simulink model "SIL_Microgrid"  (R2024a)
settings: Solver=FixedStepDiscrete  StartTime=0.0  StopTime=10  FixedStep=T_simulation  RelTol=1e-3
model workspace (MAT data in the model file):
  ICAR = 3200
  ICR = 3200
  P_0 = 0
  P_s = 10000
  Q_0 = 0
  Q_s = 1000
  T_f_VI = 0.1
  T_sampleFFR = 0.01
  T_simulation = 0.001
  batteryCellCapacity_Ah = 2
  m_p_VI = 0.1
  numberCellsParallel = 1
  numberCellsSerial = 200
libraries: spsControlledCurrentSourceLib x6, spsThreePhaseVIMeasurementLib x4, spsControlledVoltageSourceLib x3, spsGroundLib x3, spsThreePhaseParallelRLCBranchLib x3, spsThreePhaseSeriesRLCBranchLib x3, eeGeneralControl x2, simulink_extras x2, spsThreePhaseSineGeneratorLib x2, eeSinGeneratorThreePhase x1, eePowerMeasurement x1, sps_lib x1
(part 1 of 2)
settings Model: Creator=Jonathan  LastModifiedBy=Jonathan
settings DebuggingCC: AlgebraicLoopMsg=none

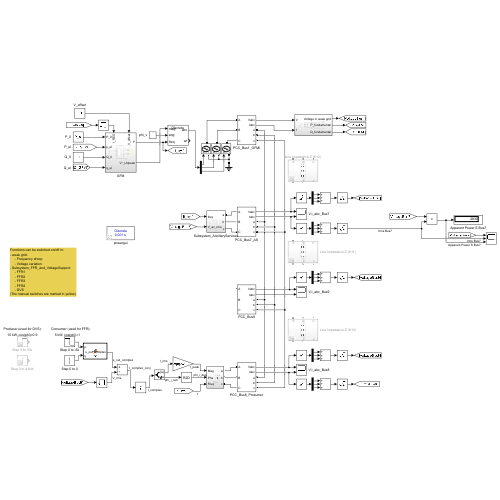
[thumbnail: Simulink's stored preview of the top-level diagram]
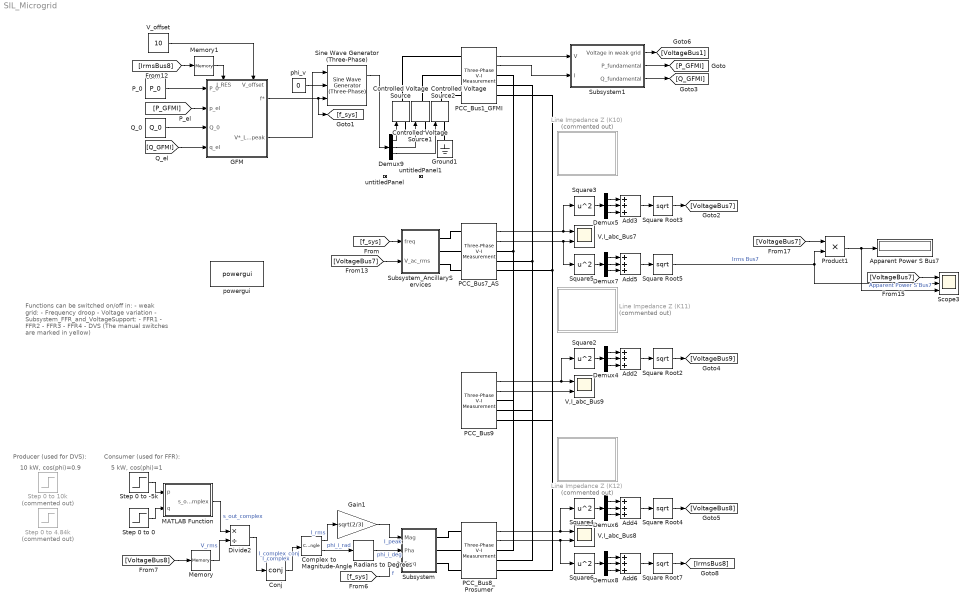
== system SIL_Microgrid ==
  note: Producer (used for DVS):
  note: 5 kW, cos(phi)=1
  note: Functions can be switched on/off in:
      | - weak grid:
      |      - Frequency droop
      |      - Voltage variation
      | - Subsystem_FFR_and_VoltageSupport:
      |      - FFR1
      |      - FFR2
      |      - FFR3
      |      - FFR4
      |      - DVS
      | (The manual switches are marked in yellow)
  note: 10 kW, cos(phi)=0.9
  note: Consumer (used for FFR):
  Add{2..6} (5 alike) : Sum  Inputs=+++
  Apparent Power S Bus7 : Display
  Complex to Magnitude-Angle : ComplexToMagnitudeAngle
  Conj : Math  Operator=conj
  Controlled Voltage Source : spsControlledVoltageSourceLib/Controlled Voltage Source  Initialize=on  Source_Type=AC  Amplitude=326.6  Phase=0  Frequency=50  Measurements=None
  Controlled Voltage Source1 : spsControlledVoltageSourceLib/Controlled Voltage Source  Initialize=on  Source_Type=AC  Amplitude=326.6  Phase=-120  Frequency=50  Measurements=None
  Controlled Voltage Source2 : spsControlledVoltageSourceLib/Controlled Voltage Source  Initialize=on  Source_Type=AC  Amplitude=326.6  Phase=120  Frequency=50  Measurements=None
  Demux{4..9} (6 alike) : Demux  Outputs=3
  Divide2 : Product  Inputs=*/
  GFM : Subsystem
      settings: PortSchema="{\"entries\":[{\"content\":{\"sides\":[{\"content\":{\"connectorIds\":[\"In1\",\"In2\",\"In3\",\"In4\"]},\"type\":\"ConnectorPlacement.EquallySpacedRectSide\",\"uuid\":\"70744577-9cbd-485e-8d22-2cdc6614abc5\"},{\"content\":{\"connectorIds\":[\"Out1\",\"Out2\"],\"side\":\"RIGHT\"},\"type\":\"ConnectorPlacement.EquallySpacedRectSide\",\"uuid\":\"2f581cd8-3e99-41c2-bd25-93a3cdbcfefe\"},{\"content\":{\"connectorIds\":[\"In5\",\"In6\"],\"side\":\"TOP\"},\"type\":\"ConnectorPlacement.EquallySpacedRectSide\",\"uuid\":\"2438c3ee-2e6d-4bc7-8ab2-fb42a3d6bd8d\"}]},\"type\":\"ConnectorPlacement.EquallySpacedConnector\",\"uuid\":\"f616edec-0a6a-4344-b22a-63fd0f376dec\"}],\"packageUris\":[\"http://schema.mathworks.com/mf0/Connector/R2020b\"],\"version\":\"1.0\"}"
  Gain1 : Gain  Gain=sqrt(2/3)
  Ground1 : spsGroundLib/Ground  LConnTagsString=a
  Line Impedance Z (K10) : Subsystem  Commented=on
      settings: PortSchema="{\"entries\":[{\"content\":{\"sides\":[{\"content\":{},\"type\":\"ConnectorPlacement.EquallySpacedRectSide\",\"uuid\":\"967be372-6ccd-4927-ad63-8f64c52d0a23\"},{\"content\":{\"side\":\"RIGHT\"},\"type\":\"ConnectorPlacement.EquallySpacedRectSide\",\"uuid\":\"6c6d6daf-7e7b-4653-bd63-75b84b3ffee7\"},{\"content\":{\"connectorIds\":[\"LConn1\",\"LConn2\",\"LConn3\"],\"side\":\"TOP\"},\"type\":\"ConnectorPlacement.EquallySpacedRectSide\",\"uuid\":\"f177627f-2459-471a-b373-8b10aeb44ac5\"},{\"content\":{\"connectorIds\":[\"RConn1\",\"RConn2\",\"RConn3\"],\"side\":\"BOTTOM\"},\"type\":\"ConnectorPlacement.EquallySpacedRectSide\",\"uuid\":\"e0b4a5a7-f3ab-42c0-b577-2901c408a3bd\"}]},\"type\":\"ConnectorPlacement.EquallySpacedConnector\",\"uuid\":\"27af90a7-8748-4802-82c9-fad952d81430\"}],\"packageUris\":[\"http://schema.mathworks.com/mf0/Connector/R2020b\"],\"version\":\"1.0\"}"
  Line Impedance Z (K11) : Subsystem  Commented=on
      settings: PortSchema="{\"entries\":[{\"content\":{\"sides\":[{\"content\":{},\"type\":\"ConnectorPlacement.EquallySpacedRectSide\",\"uuid\":\"967be372-6ccd-4927-ad63-8f64c52d0a23\"},{\"content\":{\"side\":\"RIGHT\"},\"type\":\"ConnectorPlacement.EquallySpacedRectSide\",\"uuid\":\"6c6d6daf-7e7b-4653-bd63-75b84b3ffee7\"},{\"content\":{\"connectorIds\":[\"LConn1\",\"LConn2\",\"LConn3\"],\"side\":\"TOP\"},\"type\":\"ConnectorPlacement.EquallySpacedRectSide\",\"uuid\":\"f177627f-2459-471a-b373-8b10aeb44ac5\"},{\"content\":{\"connectorIds\":[\"RConn1\",\"RConn2\",\"RConn3\"],\"side\":\"BOTTOM\"},\"type\":\"ConnectorPlacement.EquallySpacedRectSide\",\"uuid\":\"e0b4a5a7-f3ab-42c0-b577-2901c408a3bd\"}]},\"type\":\"ConnectorPlacement.EquallySpacedConnector\",\"uuid\":\"27af90a7-8748-4802-82c9-fad952d81430\"}],\"packageUris\":[\"http://schema.mathworks.com/mf0/Connector/R2020b\"],\"version\":\"1.0\"}"
  Line Impedance Z (K12) : Subsystem  Commented=on
      settings: PortSchema="{\"entries\":[{\"content\":{\"sides\":[{\"content\":{},\"type\":\"ConnectorPlacement.EquallySpacedRectSide\",\"uuid\":\"967be372-6ccd-4927-ad63-8f64c52d0a23\"},{\"content\":{\"side\":\"RIGHT\"},\"type\":\"ConnectorPlacement.EquallySpacedRectSide\",\"uuid\":\"6c6d6daf-7e7b-4653-bd63-75b84b3ffee7\"},{\"content\":{\"connectorIds\":[\"LConn1\",\"LConn2\",\"LConn3\"],\"side\":\"TOP\"},\"type\":\"ConnectorPlacement.EquallySpacedRectSide\",\"uuid\":\"f177627f-2459-471a-b373-8b10aeb44ac5\"},{\"content\":{\"connectorIds\":[\"RConn1\",\"RConn2\",\"RConn3\"],\"side\":\"BOTTOM\"},\"type\":\"ConnectorPlacement.EquallySpacedRectSide\",\"uuid\":\"e0b4a5a7-f3ab-42c0-b577-2901c408a3bd\"}]},\"type\":\"ConnectorPlacement.EquallySpacedConnector\",\"uuid\":\"27af90a7-8748-4802-82c9-fad952d81430\"}],\"packageUris\":[\"http://schema.mathworks.com/mf0/Connector/R2020b\"],\"version\":\"1.0\"}"
  MATLAB Function : MATLAB Function  TreatAsAtomicUnit=on
  Memory : Memory  InitialCondition=400
  Memory1 : Memory
  PCC_Bus1_GFMI : spsThreePhaseVIMeasurementLib/Three-Phase V-I Measurement  VoltageMeasurement=phase-to-ground  SetLabelV=off  LabelV=Vabc  Vpu=off  VpuLL=off  CurrentMeasurement=yes  SetLabelI=off  LabelI=Iabc  Ipu=off  Pbase=100e6  Vbase=500e3  OutputType=Complex  PhasorSimulation=off  PSBequivalent=0
  PCC_Bus7_AS : spsThreePhaseVIMeasurementLib/Three-Phase V-I Measurement  VoltageMeasurement=phase-to-ground  SetLabelV=off  LabelV=Vabc  Vpu=off  VpuLL=off  CurrentMeasurement=yes  SetLabelI=off  LabelI=Iabc  Ipu=off  Pbase=100e6  Vbase=500e3  OutputType=Complex  PhasorSimulation=off  PSBequivalent=0
  PCC_Bus8_Prosumer : spsThreePhaseVIMeasurementLib/Three-Phase V-I Measurement  VoltageMeasurement=phase-to-ground  SetLabelV=off  LabelV=Vabc  Vpu=off  VpuLL=off  CurrentMeasurement=yes  SetLabelI=off  LabelI=Iabc  Ipu=off  Pbase=100e6  Vbase=500e3  OutputType=Complex  PhasorSimulation=off  PSBequivalent=0
  PCC_Bus9 : spsThreePhaseVIMeasurementLib/Three-Phase V-I Measurement  VoltageMeasurement=phase-to-ground  SetLabelV=off  LabelV=Vabc  Vpu=off  VpuLL=off  CurrentMeasurement=yes  SetLabelI=off  LabelI=Iabc  Ipu=off  Pbase=100e6  Vbase=500e3  OutputType=Complex  PhasorSimulation=off  PSBequivalent=0
  P_0 : Constant  Value=P_0
  Product1 : Product
  Q_0 : Constant  Value=Q_0
  Radians to Degrees : simulink_extras/Transformations/Radians to Degrees
  Scope3 : Scope  NumInputPorts=3
  Sine Wave Generator (Three-Phase) : eeSinGeneratorThreePhase/Sine Wave Generator (Three-Phase)  Ts=-1
      settings: LibrarySourceBlock=|
      | ee_sl_lib/General Control/Sine Wave Generator
      | (Three-Phase)
  Square Root{2..5,7} (5 alike) : Sqrt  OutputSignalType=real
  Square{2..6} (5 alike) : Math  Operator=square  OutputSignalType=real
  Step 0 to -5k : Step  Time=0.5  Before=P_0  After=-5e3  SampleTime=0
  Step 0 to 0 : Step  Time=0.5  After=0  SampleTime=0
  Step 0 to 10k : Step  Commented=on  Time=0.5  After=10e3  SampleTime=0
  Step 0 to 4.84k : Step  Commented=on  Time=0.5  After=4.84e3  SampleTime=0
  Subsystem : Subsystem
  Subsystem1 : Subsystem
  Subsystem_AncillaryServices : Subsystem
  V,I_abc_Bus7 : Scope  NumInputPorts=2
  V,I_abc_Bus8 : Scope  NumInputPorts=2
  V,I_abc_Bus9 : Scope  NumInputPorts=2
  V_offset : Constant  Value=10
  phi_v : Constant  Value=0
  powergui : sps_lib/powergui  Priority=1  SimulationMode=Discrete  SampleTime=T_simulation  frequency=50  Iterations=50  frequencyindice=50  Pbase=100e6  ErrMax=1e-4  UnitsV=kV  UnitsW=MW  buscounter=0  FunctionMessages=off  echomessages=off  EnableUseOfTLC=off  CurrentSourceSwitches=off  DisableSnubberDevices=off  DisableRonSwitches=off  DisableVfSwitches=off  DisplayEquations=off  AutomaticDiscreteSolvers=off  SolverType=Tustin/Backward Euler (TBE)  Interpol=off  ExternalGateDelay=off  methode=off  Ts=100  x0status=blocks  SPID=on  SwTol=0  HookPort=off  NonlinearTolerance=1e-4  nMaxIteration=100  ContinueOnMaxIteration=off  RestoreLinks=warning  ResistiveCurrentMeasurement=off  Frange=[0:2:500]  Ylog=off  Xlog=on  ShowGrid=off  save=off  variable=ZData  structure=0  ZoomFFT=off  StartTime=0.0  cycles=1  DisplayStyle=1  fundamental=60  FreqAxis=off  MaxFrequency=1000  frequencyindicesteady=1  RmsSteady=1  display=off
  untitledPanel : Subsystem  Tag=HiddenForWebPanel  IsWebBlockPanel=on
  untitledPanel1 : Subsystem  Tag=HiddenForWebPanel  IsWebBlockPanel=on
  wires:
  PCC_Bus9/1 -> V,I_abc_Bus9/1, Square2/1
  PCC_Bus9/2 -> V,I_abc_Bus9/2
  P_0/1 -> GFM/1(P_0)
  [P_GFMI] -> GFM/2(p_el)
  [Q_GFMI] -> GFM/4(q_el)
  PCC_Bus7_AS/1 -> Square3/1, V,I_abc_Bus7/1
  Square Root2/1 -> [VoltageBus9]
  Demux4/2 -> Add2/2
  Square2/1 -> Demux4/1
  Demux4/1 -> Add2/1
  Add2/1 -> Square Root2/1
  Demux4/3 -> Add2/3
  Square3/1 -> Demux5/1
  Demux5/2 -> Add3/2
  Add3/1 -> Square Root3/1
  Demux5/1 -> Add3/1
  Demux5/3 -> Add3/3
  Square Root4/1 -> [VoltageBus8]
  Demux6/1 -> Add4/1
  Demux6/2 -> Add4/2
  Demux6/3 -> Add4/3
  Square4/1 -> Demux6/1
  Add4/1 -> Square Root4/1
  PCC_Bus8_Prosumer/1 -> V,I_abc_Bus8/1, Square4/1
  [f_sys] -> Subsystem/3(Freq)  "f"
  Gain1/1 -> Subsystem/1(Mag)  "I_peak"
  Add5/1 -> Square Root5/1
  Square Root3/1 -> [VoltageBus7]
  Demux7/3 -> Add5/3
  Demux7/1 -> Add5/1
  Square5/1 -> Demux7/1
  Demux7/2 -> Add5/2
  PCC_Bus7_AS/2 -> Square5/1, V,I_abc_Bus7/2
  Product1/1 -> Scope3/3, Apparent Power S Bus7/1  "Apparent Power S Bus7"
  Square Root5/1 -> Product1/2, Scope3/2  "Irms Bus7"
  [f_sys] -> Subsystem_AncillaryServices/1(freq)
  Q_0/1 -> GFM/3(Q_0)
  V_offset/1 -> GFM/6(V_offset)
  Divide2/1 -> Conj/1  "I_complex_conj"
  Radians to Degrees/1 -> Subsystem/2(Pha)  "phi_i_deg"
  MATLAB Function/1(s_out_complex) -> Divide2/1  "s_out_complex"
  Complex to Magnitude-Angle/1 -> Gain1/1  "I_rms"
  [VoltageBus8] -> Memory/1
  Complex to Magnitude-Angle/2 -> Radians to Degrees/1  "phi_i_rad"
  Conj/1 -> Complex to Magnitude-Angle/1  "I_complex"
  Step 0 to -5k/1 -> MATLAB Function/1(p)
  Step 0 to 0/1 -> MATLAB Function/2(q)
  Memory/1 -> Divide2/2  "V_rms"
  Demux8/3 -> Add6/3
  Square6/1 -> Demux8/1
  Add6/1 -> Square Root7/1
  Demux8/2 -> Add6/2
  Demux8/1 -> Add6/1
  Square Root7/1 -> [IrmsBus8]
  [IrmsBus8] -> Memory1/1
  PCC_Bus8_Prosumer/2 -> V,I_abc_Bus8/2, Square6/1
  [VoltageBus7] -> Subsystem_AncillaryServices/2(V_ac_rms)
  Demux9/1 -> Controlled Voltage Source/1
  Sine Wave Generator (Three-Phase)/1 -> Demux9/1
  Demux9/2 -> Controlled Voltage Source1/1
  Demux9/3 -> Controlled Voltage Source2/1
  phi_v/1 -> Sine Wave Generator (Three-Phase)/2
  GFM/1(f*) -> [f_sys], Sine Wave Generator (Three-Phase)/3
  GFM/2(V*_LNpeak) -> Sine Wave Generator (Three-Phase)/1
  Memory1/1 -> GFM/5(I_RES)
  Subsystem1/2(P_fundamental) -> [P_GFMI]
  PCC_Bus1_GFMI/1 -> Subsystem1/1(V)
  PCC_Bus1_GFMI/2 -> Subsystem1/2(I)
  Subsystem1/1(Voltage in weak grid) -> [VoltageBus1]
  Subsystem1/3(Q_fundamental) -> [Q_GFMI]
  [VoltageBus7] -> Product1/1
  [VoltageBus7] -> Scope3/1
  connections:
  PCC_Bus8_Prosumer/RConn2 -- PCC_Bus9/RConn2 -- PCC_Bus1_GFMI/RConn2 -- PCC_Bus7_AS/RConn2
  PCC_Bus8_Prosumer/RConn1 -- PCC_Bus9/RConn1 -- PCC_Bus1_GFMI/RConn1 -- PCC_Bus7_AS/RConn1
  PCC_Bus8_Prosumer/RConn3 -- PCC_Bus9/RConn3 -- PCC_Bus1_GFMI/RConn3 -- PCC_Bus7_AS/RConn3
  Subsystem_AncillaryServices/RConn2 -- PCC_Bus7_AS/LConn2
  Subsystem_AncillaryServices/RConn1 -- PCC_Bus7_AS/LConn1
  Subsystem_AncillaryServices/RConn3 -- PCC_Bus7_AS/LConn3
  Subsystem/RConn2 -- PCC_Bus8_Prosumer/LConn2
  Subsystem/RConn1 -- PCC_Bus8_Prosumer/LConn1
  Subsystem/RConn3 -- PCC_Bus8_Prosumer/LConn3
  Controlled Voltage Source2/RConn1 -- PCC_Bus1_GFMI/LConn3
  Controlled Voltage Source/RConn1 -- PCC_Bus1_GFMI/LConn1
  Controlled Voltage Source1/RConn1 -- PCC_Bus1_GFMI/LConn2
  Ground1/LConn1 -- Controlled Voltage Source/LConn1 -- Controlled Voltage Source1/LConn1 -- Controlled Voltage Source2/LConn1

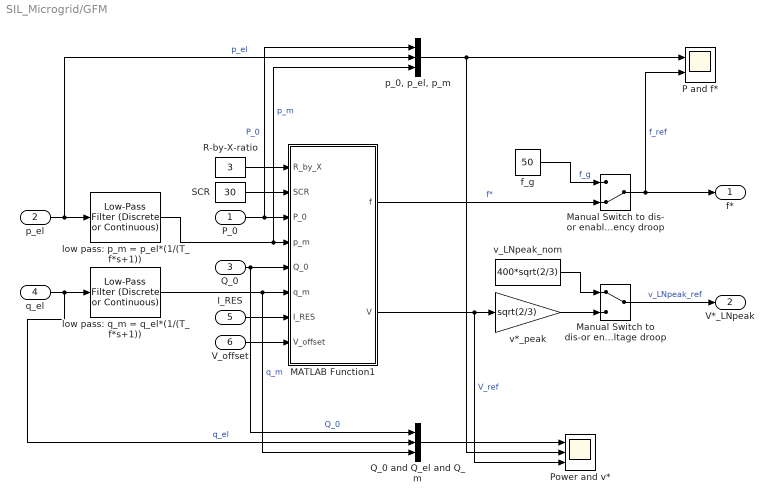
== system SIL_Microgrid/GFM ==
  P_0 : Inport
  p_el : Inport  Port=2
  Q_0 : Inport  Port=3
  q_el : Inport  Port=4
  I_RES : Inport  Port=5
  V_offset : Inport  Port=6
  MATLAB Function1 : MATLAB Function  TreatAsAtomicUnit=on
  Manual Switch to dis- or enable frequency droop : ManualSwitch  CurrentSetting=0
  Manual Switch to dis-or enable voltage droop : ManualSwitch
  P and f* : Scope  NumInputPorts=2
  Power and v* : Scope  NumInputPorts=3
  Q_0 and Q_el and Q_m : Mux  Inputs=3
  R-by-X-ratio : Constant  Value=3
  SCR : Constant  Value=30
  f_g : Constant  Value=50
  low pass: p_m = p_el*(1/(T_f*s+1)) : eeGeneralControl/Low-Pass Filter (Discrete or Continuous)  K=1  T=0.05  B=inf  A=-inf  init_option=Specify as parameter  x0=P_0  Ts=-1
  low pass: q_m = q_el*(1/(T_f*s+1)) : eeGeneralControl/Low-Pass Filter (Discrete or Continuous)  K=1  T=0.1  B=inf  A=-inf  init_option=Specify as parameter  x0=Q_0+Q_s-1006  Ts=-1
  "p_0, p_el, p_m" : Mux  Inputs=3
  v*_peak : Gain  Gain=sqrt(2/3)
  v_LNpeak_nom : Constant  Value=400*sqrt(2/3)
  f* : Outport
  V*_LNpeak : Outport  Port=2
  wires:
  p_el/1 -> low pass: p_m = p_el*(1/(T_f*s+1))/1, "p_0, p_el, p_m"/2  "p_el"
  f_g/1 -> Manual Switch to dis- or enable frequency droop/1  "f_g"
  low pass: p_m = p_el*(1/(T_f*s+1))/1 -> "p_0, p_el, p_m"/3, MATLAB Function1/4(p_m)  "p_m"
  P_0/1 -> MATLAB Function1/3(P_0), "p_0, p_el, p_m"/1  "P_0"
  "p_0, p_el, p_m"/1 -> Power and v*/2, P and f*/1
  Q_0/1 -> Q_0 and Q_el and Q_m/1, MATLAB Function1/5(Q_0)  "Q_0"
  low pass: q_m = q_el*(1/(T_f*s+1))/1 -> Q_0 and Q_el and Q_m/3, MATLAB Function1/6(q_m)  "q_m"
  q_el/1 -> Q_0 and Q_el and Q_m/2, low pass: q_m = q_el*(1/(T_f*s+1))/1  "q_el"
  v_LNpeak_nom/1 -> Manual Switch to dis-or enable voltage droop/1
  Q_0 and Q_el and Q_m/1 -> Power and v*/1
  Manual Switch to dis- or enable frequency droop/1 -> P and f*/2, f*/1  "f_ref"
  v*_peak/1 -> Manual Switch to dis-or enable voltage droop/2
  Manual Switch to dis-or enable voltage droop/1 -> V*_LNpeak/1  "v_LNpeak_ref"
  SCR/1 -> MATLAB Function1/2(SCR)
  R-by-X-ratio/1 -> MATLAB Function1/1(R_by_X)
  MATLAB Function1/1(f) -> Manual Switch to dis- or enable frequency droop/2  "f*"
  MATLAB Function1/2(V) -> v*_peak/1, Power and v*/3  "V_ref"
  V_offset/1 -> MATLAB Function1/8(V_offset)
  I_RES/1 -> MATLAB Function1/7(I_RES)

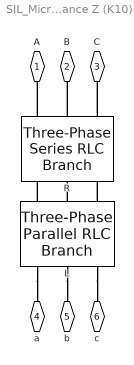
== system SIL_Microgrid/Line Impedance Z (K10) ==
  L : spsThreePhaseParallelRLCBranchLib/Three-Phase Parallel RLC Branch  LConnTagsString=A|B|C  RConnTagsString=A|B|C  BranchType=RL  Resistance=1e6  Inductance=3e-5  Capacitance=1e-6  Measurements=None
  R : spsThreePhaseSeriesRLCBranchLib/Three-Phase Series RLC Branch  LConnTagsString=A|B|C  RConnTagsString=A|B|C  BranchType=R  Resistance=0.03087  Inductance=1e-3  Capacitance=1e-6  Measurements=Branch voltages and currents
  A : PMIOPort  Side=Left
  B : PMIOPort  Port=2  Side=Left
  C : PMIOPort  Port=3  Side=Left
  a : PMIOPort  Port=4  Side=Right
  b : PMIOPort  Port=5  Side=Right
  c : PMIOPort  Port=6  Side=Right
  connections:
  L/RConn3 -- c/RConn1
  R/LConn1 -- A/RConn1
  L/LConn1 -- R/RConn1
  L/LConn2 -- R/RConn2
  R/LConn3 -- C/RConn1
  L/LConn3 -- R/RConn3
  L/RConn1 -- a/RConn1
  R/LConn2 -- B/RConn1
  L/RConn2 -- b/RConn1

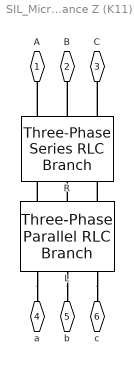
== system SIL_Microgrid/Line Impedance Z (K11) ==
  L : spsThreePhaseParallelRLCBranchLib/Three-Phase Parallel RLC Branch  LConnTagsString=A|B|C  RConnTagsString=A|B|C  BranchType=RL  Resistance=1e6  Inductance=2.14e-5  Capacitance=1e-6  Measurements=None
  R : spsThreePhaseSeriesRLCBranchLib/Three-Phase Series RLC Branch  LConnTagsString=A|B|C  RConnTagsString=A|B|C  BranchType=R  Resistance=0.02179  Inductance=1e-3  Capacitance=1e-6  Measurements=Branch voltages and currents
  A : PMIOPort  Side=Left
  B : PMIOPort  Port=2  Side=Left
  C : PMIOPort  Port=3  Side=Left
  a : PMIOPort  Port=4  Side=Right
  b : PMIOPort  Port=5  Side=Right
  c : PMIOPort  Port=6  Side=Right
  connections:
  L/RConn2 -- b/RConn1
  R/LConn2 -- B/RConn1
  L/RConn1 -- a/RConn1
  L/LConn3 -- R/RConn3
  R/LConn3 -- C/RConn1
  L/LConn2 -- R/RConn2
  L/LConn1 -- R/RConn1
  R/LConn1 -- A/RConn1
  L/RConn3 -- c/RConn1

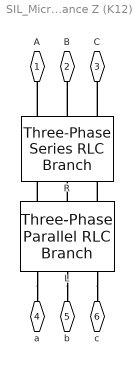
== system SIL_Microgrid/Line Impedance Z (K12) ==
  L : spsThreePhaseParallelRLCBranchLib/Three-Phase Parallel RLC Branch  LConnTagsString=A|B|C  RConnTagsString=A|B|C  BranchType=RL  Resistance=1e6  Inductance=2.14e-5  Capacitance=1e-6  Measurements=None
  R : spsThreePhaseSeriesRLCBranchLib/Three-Phase Series RLC Branch  LConnTagsString=A|B|C  RConnTagsString=A|B|C  BranchType=R  Resistance=0.02179  Inductance=1e-3  Capacitance=1e-6  Measurements=Branch voltages and currents
  A : PMIOPort  Side=Left
  B : PMIOPort  Port=2  Side=Left
  C : PMIOPort  Port=3  Side=Left
  a : PMIOPort  Port=4  Side=Right
  b : PMIOPort  Port=5  Side=Right
  c : PMIOPort  Port=6  Side=Right
  connections:
  L/RConn3 -- c/RConn1
  R/LConn1 -- A/RConn1
  L/LConn1 -- R/RConn1
  L/LConn2 -- R/RConn2
  R/LConn3 -- C/RConn1
  L/LConn3 -- R/RConn3
  L/RConn1 -- a/RConn1
  R/LConn2 -- B/RConn1
  L/RConn2 -- b/RConn1

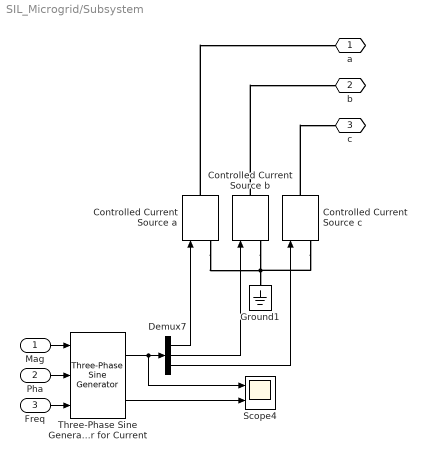
== system SIL_Microgrid/Subsystem ==
  Mag : Inport
  Pha : Inport  Port=2
  Freq : Inport  Port=3
  Controlled Current Source a : spsControlledCurrentSourceLib/Controlled Current Source  Initialize=on  Source_Type=AC  Amplitude=0  Phase=0  Frequency=50  Measurements=Current
  Controlled Current Source b : spsControlledCurrentSourceLib/Controlled Current Source  Initialize=on  Source_Type=AC  Amplitude=0  Phase=-120  Frequency=50  Measurements=Current
  Controlled Current Source c : spsControlledCurrentSourceLib/Controlled Current Source  Initialize=on  Source_Type=AC  Amplitude=0  Phase=120  Frequency=50  Measurements=Current
  Demux7 : Demux  Outputs=3
  Ground1 : spsGroundLib/Ground  LConnTagsString=a
  Scope4 : Scope  NumInputPorts=2
  Three-Phase Sine Generator for Current : spsThreePhaseSineGeneratorLib/Three-Phase Sine Generator  Ts=T_simulation
      settings: LibrarySourceBlock=|
      | sps_lib/Sources/Signal Generator Sources/Three-Phase
      | Sine Generator
  a : PMIOPort  Side=Right
  b : PMIOPort  Port=2  Side=Right
  c : PMIOPort  Port=3  Side=Right
  wires:
  Demux7/3 -> Controlled Current Source c/1
  Three-Phase Sine Generator for Current/1 -> Scope4/1, Demux7/1
  Demux7/2 -> Controlled Current Source b/1
  Demux7/1 -> Controlled Current Source a/1
  Three-Phase Sine Generator for Current/2 -> Scope4/2
  Mag/1 -> Three-Phase Sine Generator for Current/1
  Freq/1 -> Three-Phase Sine Generator for Current/3
  Pha/1 -> Three-Phase Sine Generator for Current/2
  connections:
  Controlled Current Source c/RConn1 -- c/RConn1
  Ground1/LConn1 -- Controlled Current Source c/LConn1 -- Controlled Current Source a/LConn1 -- Controlled Current Source b/LConn1
  Controlled Current Source b/RConn1 -- b/RConn1
  Controlled Current Source a/RConn1 -- a/RConn1

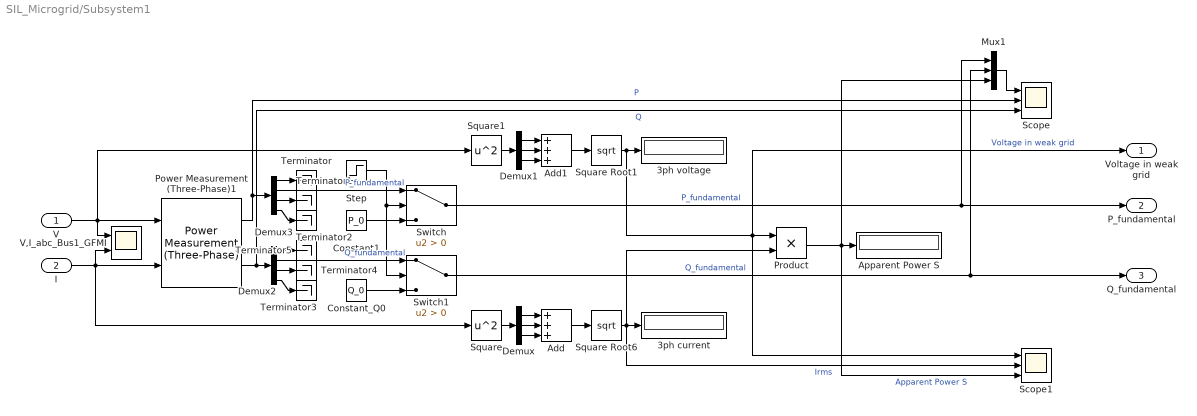
== system SIL_Microgrid/Subsystem1 ==
  V : Inport
  I : Inport  Port=2
  3ph current : Display
  3ph voltage : Display
  Add : Sum  Inputs=+++
  Add1 : Sum  Inputs=+++
  Apparent Power S : Display
  Constant1 : Constant  Value=P_0
  Constant_Q0 : Constant  Value=Q_0
  Demux : Demux  Outputs=3
  Demux1 : Demux  Outputs=3
  Demux2 : Demux
  Demux3 : Demux
  Mux1 : Mux  Inputs=3
  Power Measurement (Three-Phase)1 : eePowerMeasurement/Power Measurement (Three-Phase)  LabelModeActiveChoice=Discrete  F=50  K=[0 1 2 3]  Seq=Positive  Ts=T_simulation
  Product : Product
  Scope : Scope  NumInputPorts=3
  Scope1 : Scope  NumInputPorts=3
  Square : Math  Operator=square  OutputSignalType=real
  Square Root1 : Sqrt  OutputSignalType=real
  Square Root6 : Sqrt  OutputSignalType=real
  Square1 : Math  Operator=square  OutputSignalType=real
  Step : Step  Time=1/50  SampleTime=0
  Switch : Switch  Criteria=u2 > Threshold  SaturateOnIntegerOverflow=off  InputSameDT=off
  Switch1 : Switch  Criteria=u2 > Threshold  SaturateOnIntegerOverflow=off  InputSameDT=off
  Terminator{,1..5} (6 alike) : Terminator
  V,I_abc_Bus1_GFMI : Scope  NumInputPorts=2
  Voltage in weak grid : Outport
  P_fundamental : Outport  Port=2
  Q_fundamental : Outport  Port=3
  wires:
  Switch1/1 -> Q_fundamental/1, Mux1/2  "Q_fundamental"
  Demux3/3 -> Terminator1/1
  Demux1/3 -> Add1/3
  V/1 -> V,I_abc_Bus1_GFMI/1, Square1/1, Power Measurement (Three-Phase)1/1
  Demux1/1 -> Add1/1
  Square Root6/1 -> Product/2, Scope1/2, 3ph current/1  "Irms"
  Switch/1 -> Mux1/1, P_fundamental/1  "P_fundamental"
  Constant1/1 -> Switch/3
  Demux3/2 -> Switch/1  "P_fundamental"
  Demux/2 -> Add/2
  Add/1 -> Square Root6/1
  Square Root1/1 -> Voltage in weak grid/1, Scope1/1, Product/1, 3ph voltage/1  "Voltage in weak grid"
  Product/1 -> Mux1/3, Apparent Power S/1, Scope1/3  "Apparent Power S"
  Demux2/3 -> Terminator4/1
  Power Measurement (Three-Phase)1/1 -> Scope/2, Demux3/1  "P"
  Square1/1 -> Demux1/1
  Demux1/2 -> Add1/2
  Step/1 -> Switch1/2, Switch/2
  I/1 -> Square/1, V,I_abc_Bus1_GFMI/2, Power Measurement (Three-Phase)1/2
  Add1/1 -> Square Root1/1
  Demux/1 -> Add/1
  Power Measurement (Three-Phase)1/2 -> Scope/3, Demux2/1  "Q"
  Demux3/4 -> Terminator2/1
  Demux/3 -> Add/3
  Mux1/1 -> Scope/1
  Constant_Q0/1 -> Switch1/3
  Demux2/2 -> Switch1/1  "Q_fundamental"
  Square/1 -> Demux/1
  Demux2/4 -> Terminator3/1
  Demux3/1 -> Terminator/1
  Demux2/1 -> Terminator5/1

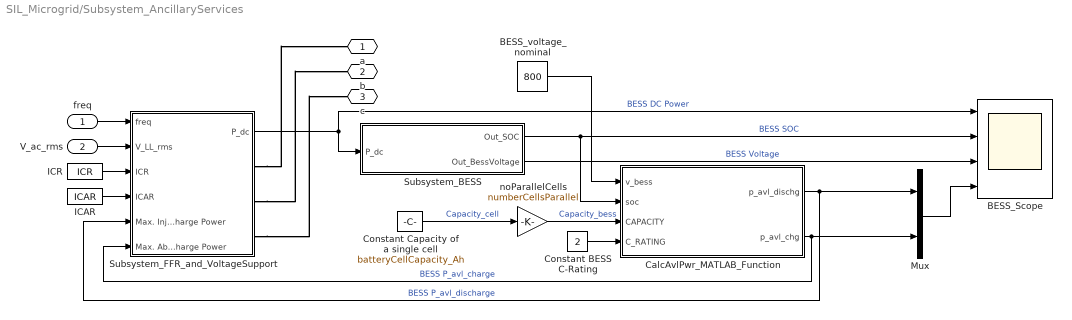
== system SIL_Microgrid/Subsystem_AncillaryServices ==
  freq : Inport
  V_ac_rms : Inport  Port=2
  BESS_Scope : Scope  NumInputPorts=4
  BESS_voltage_nominal : Constant  Value=800
  CalcAvlPwr_MATLAB_Function : MATLAB Function  TreatAsAtomicUnit=on
  Constant BESS C-Rating : Constant  Value=2
  Constant Capacity of a single cell : Constant  Value=batteryCellCapacity_Ah
  ICAR : Constant  Value=ICAR
  ICR : Constant  Value=ICR
  Mux : Mux  Inputs=2
  Subsystem_BESS : Subsystem
  Subsystem_FFR_and_VoltageSupport : Subsystem  SystemSampleTime=1e-2
  noParallelCells : Gain  Gain=numberCellsParallel
  a : PMIOPort  Side=Right
  b : PMIOPort  Port=2  Side=Right
  c : PMIOPort  Port=3  Side=Right
  wires:
  CalcAvlPwr_MATLAB_Function/2(p_avl_chg) -> Subsystem_FFR_and_VoltageSupport/6(Max. Absorption/Charge Power), Mux/2  "BESS P_avl_charge"
  Subsystem_FFR_and_VoltageSupport/1(P_dc) -> Subsystem_BESS/1(P_dc), BESS_Scope/1  "BESS DC Power"
  noParallelCells/1 -> CalcAvlPwr_MATLAB_Function/3(CAPACITY)  "Capacity_bess"
  Subsystem_BESS/2(Out_BessVoltage) -> BESS_Scope/3  "BESS Voltage"
  Constant BESS C-Rating/1 -> CalcAvlPwr_MATLAB_Function/4(C_RATING)
  ICAR/1 -> Subsystem_FFR_and_VoltageSupport/4(ICAR)
  ICR/1 -> Subsystem_FFR_and_VoltageSupport/3(ICR)
  Mux/1 -> BESS_Scope/4
  freq/1 -> Subsystem_FFR_and_VoltageSupport/1(freq)
  CalcAvlPwr_MATLAB_Function/1(p_avl_dischg) -> Subsystem_FFR_and_VoltageSupport/5(Max. Injection/Discharge Power), Mux/1  "BESS P_avl_discharge"
  Subsystem_BESS/1(Out_SOC) -> CalcAvlPwr_MATLAB_Function/2(soc), BESS_Scope/2  "BESS SOC"
  BESS_voltage_nominal/1 -> CalcAvlPwr_MATLAB_Function/1(v_bess)
  Constant Capacity of a single cell/1 -> noParallelCells/1  "Capacity_cell"
  V_ac_rms/1 -> Subsystem_FFR_and_VoltageSupport/2(V_LL_rms)
  connections:
  Subsystem_FFR_and_VoltageSupport/RConn1 -- a/RConn1
  Subsystem_FFR_and_VoltageSupport/RConn3 -- c/RConn1
  Subsystem_FFR_and_VoltageSupport/RConn2 -- b/RConn1

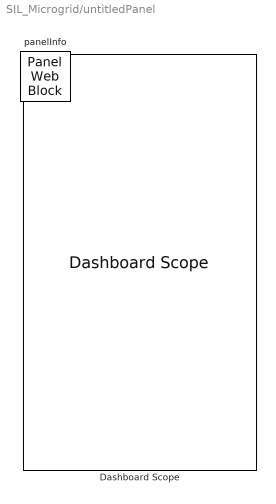
== system SIL_Microgrid/untitledPanel ==
  Dashboard Scope : DashboardScope  Tag=HiddenForWebPanel  PanelInfo="{\"height\":416,\"left\":18,\"panelId\":\"panelId-37cc0f9b-1b27-4f5b-8879-a88fc3f83368\",\"top\":18,\"type\":\"panelChild\",\"version\":\"2019b\",\"width\":233,\"zIndex\":1500002}"
  panelInfo : PanelWebBlock  Tag=HiddenForWebPanel  PanelInfo="{\"compacted\":false,\"height\":456,\"isActiveTab\":false,\"left\":1342,\"name\":\"Panel\",\"panelId\":\"panelId-37cc0f9b-1b27-4f5b-8879-a88fc3f83368\",\"popoutData\":{\"height\":602,\"left\":-529,\"maximized\":false,\"top\":114,\"width\":365},\"popoutMode\":\"windowHidden\",\"tabIndex\":0,\"tabbedSetId\":\"tabbedSet9027355487\",\"top\":39,\"type\":\"panel\",\"version\":\"2019b\",\"visible\":false,\"width\":273,\"zIndex\":1500002}"  PanelSnapshot=<binary blob, 84420 chars, not shown>

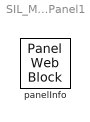
== system SIL_Microgrid/untitledPanel1 ==
  panelInfo : PanelWebBlock  Tag=HiddenForWebPanel  PanelInfo="{\"compacted\":false,\"height\":456,\"isActiveTab\":true,\"left\":1342,\"name\":\"Panel1\",\"panelId\":\"panelId-b748de57-4048-477b-a225-a0a70c3c5bc8\",\"popoutData\":{\"height\":602,\"left\":-529,\"maximized\":false,\"top\":114,\"width\":365},\"popoutMode\":\"windowHidden\",\"tabIndex\":1,\"tabbedSetId\":\"tabbedSet9027355487\",\"top\":39,\"type\":\"panel\",\"version\":\"2019b\",\"visible\":true,\"width\":273,\"zIndex\":1500004}"  PanelSnapshot=<binary blob, 5764 chars, not shown>

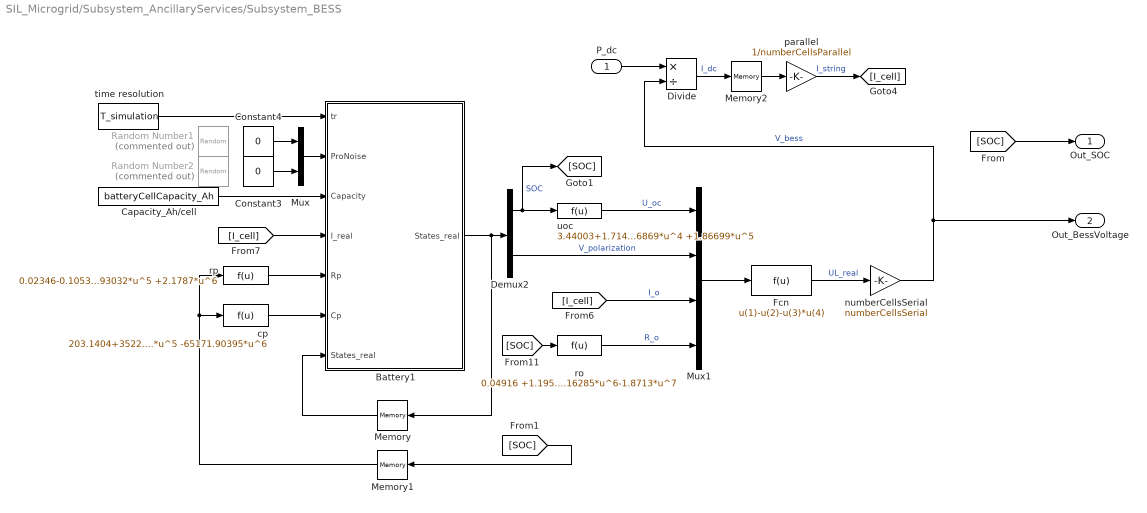
== system SIL_Microgrid/Subsystem_AncillaryServices/Subsystem_BESS ==
  P_dc : Inport
  Battery1 : MATLAB Function  TreatAsAtomicUnit=on
  Capacity_Ah/cell : Constant  Value=batteryCellCapacity_Ah
  Constant3 : Constant  Value=0
  Constant4 : Constant  Value=0
  Demux2 : Demux  Outputs=2
  Divide : Product  Inputs=*/
  Fcn : Fcn  Expr=u(1)-u(2)-u(3)*u(4)
  Memory : Memory  InitialCondition=[0.6;0]  LinearizeAsDelay=on
  Memory1 : Memory  InitialCondition=0.6  LinearizeAsDelay=on
  Memory2 : Memory
  Mux : Mux  Inputs=2
  Mux1 : Mux
  Random Number1 : RandomNumber  Commented=on  Variance=2e-8  SampleTime=5e-4
  Random Number2 : RandomNumber  Commented=on  Variance=1e-8  SampleTime=5e-4
  cp : Fcn  Expr=203.1404+3522.78847*u-31392.66753*u^2+122406.91269*u^3-227590.94382*u^4+198281.56406*u^5 -65171.90395*u^6
  numberCellsSerial : Gain  Gain=numberCellsSerial
  parallel : Gain  Gain=1/numberCellsParallel
  ro : Fcn  Expr=0.04916 +1.19552*u-6.25333*u^2+14.24181*u^3-13.93388*u^4+2.553*u^5+4.16285*u^6-1.8713*u^7
  rp : Fcn  Expr=0.02346-0.10537*u^1+1.1371*u^2-4.55188*u^3+8.26827*u^4-6.93032*u^5 +2.1787*u^6
  time resolution : Constant  Value=T_simulation
  uoc : Fcn  Expr=3.44003+1.71448*u -3.51247*u^2 +5.70868*u^3 -5.06869*u^4 +1.86699*u^5
  Out_SOC : Outport
  Out_BessVoltage : Outport  Port=2
  wires:
  Mux/1 -> Battery1/2(ProNoise)
  Fcn/1 -> numberCellsSerial/1  "UL_real"
  Memory1/1 -> cp/1, rp/1
  time resolution/1 -> Battery1/1(tr)
  Memory/1 -> Battery1/7("States_real ")
  ro/1 -> Mux1/4  "R_o"
  uoc/1 -> Mux1/1  "U_oc"
  Demux2/1 -> [SOC], uoc/1  "SOC"
  Demux2/2 -> Mux1/2  "V_polarization"
  Mux1/1 -> Fcn/1
  Constant3/1 -> Mux/2
  Constant4/1 -> Mux/1
  [I_cell] -> Mux1/3  "I_o"
  Battery1/1(States_real) -> Memory/1, Demux2/1
  rp/1 -> Battery1/5(Rp)
  cp/1 -> Battery1/6(Cp)
  Capacity_Ah/cell/1 -> Battery1/3(Capacity)
  P_dc/1 -> Divide/1
  Divide/1 -> Memory2/1  "I_dc"
  Memory2/1 -> parallel/1
  [I_cell] -> Battery1/4(I_real)
  parallel/1 -> [I_cell]  "I_string"
  numberCellsSerial/1 -> Divide/2, Out_BessVoltage/1  "V_bess"
  [SOC] -> Out_SOC/1
  [SOC] -> Memory1/1
  [SOC] -> ro/1

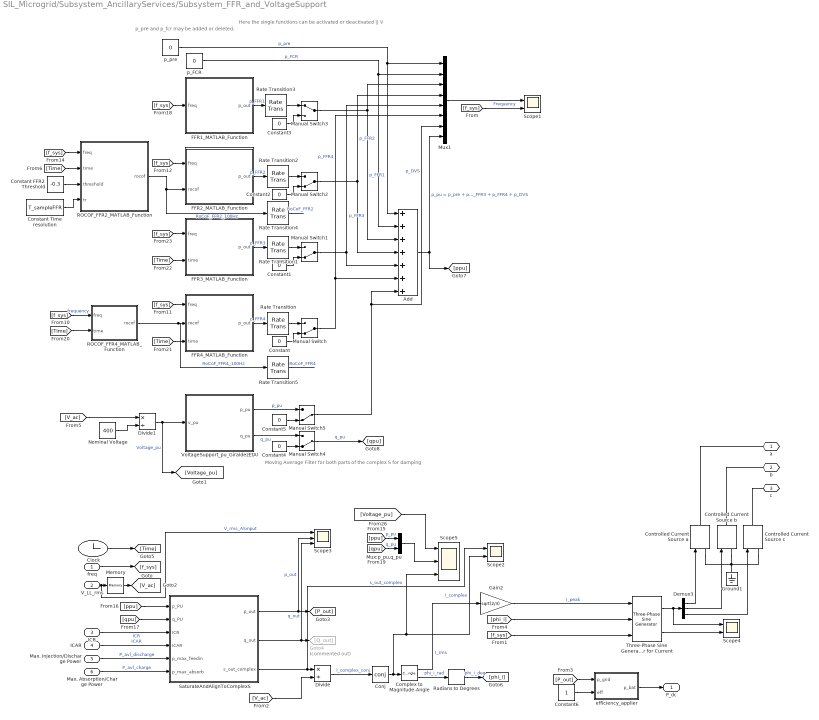
== system SIL_Microgrid/Subsystem_AncillaryServices/Subsystem_FFR_and_VoltageSupport ==
  note: Moving Average Filter for both parts of the complex S for damping
  note: Here the single functions can be activated or deactivated
      |                                                ||
      |                                                V
  note: p_pre and p_fcr may be added or deleted.
  freq : Inport
  V_LL_rms : Inport  Port=2
  ICR : Inport  Port=3
  ICAR : Inport  Port=4
  Max. Injection/Discharge Power : Inport  Port=5
  Max. Absorption/Charge Power : Inport  Port=6
  Add : Sum  Inputs=+++++++
  Clock : Clock
  Complex to Magnitude-Angle : ComplexToMagnitudeAngle
  Conj : Math  Operator=conj
  Constant{,1..5} (6 alike) : Constant  Value=0
  Constant FFR2 Threshold : Constant  Value=-0.3
  Constant Time resolution : Constant  Value=T_sampleFFR
  Constant6 : Constant
  Controlled Current Source a : spsControlledCurrentSourceLib/Controlled Current Source  Initialize=on  Source_Type=AC  Amplitude=0  Phase=0  Frequency=50  Measurements=Current
  Controlled Current Source b : spsControlledCurrentSourceLib/Controlled Current Source  Initialize=on  Source_Type=AC  Amplitude=0  Phase=-120  Frequency=50  Measurements=Current
  Controlled Current Source c : spsControlledCurrentSourceLib/Controlled Current Source  Initialize=on  Source_Type=AC  Amplitude=0  Phase=120  Frequency=50  Measurements=Current
  Demux3 : Demux  Outputs=3
  Divide : Product  Inputs=*/
  Divide1 : Product  Inputs=*/
  FFR1_MATLAB_Function : MATLAB Function  TreatAsAtomicUnit=on  SystemSampleTime=T_sampleFFR
  FFR2_MATLAB_Function : MATLAB Function  TreatAsAtomicUnit=on  SystemSampleTime=T_sampleFFR
  FFR3_MATLAB_Function : MATLAB Function  TreatAsAtomicUnit=on  SystemSampleTime=T_sampleFFR
  FFR4_MATLAB_Function : MATLAB Function  TreatAsAtomicUnit=on  SystemSampleTime=T_sampleFFR
  Gain2 : Gain  Gain=sqrt(2/3)
  Goto4 : Goto  Commented=on  GotoTag=Q_out
  Ground1 : spsGroundLib/Ground  LConnTagsString=a
  Manual Switch{,1..2,4..5} (5 alike) : ManualSwitch  CurrentSetting=0
  Manual Switch3 : ManualSwitch
  Memory : Memory  InitialCondition=400  InheritSampleTime=on
  Mux1 : Mux  Inputs=8
  Mux:p_pu,q_pu : Mux  Inputs=2
  Nominal Voltage : Constant  Value=400
  ROCOF_FFR2_MATLAB_Function : MATLAB Function  TreatAsAtomicUnit=on  SystemSampleTime=T_sampleFFR
  ROCOF_FFR4_MATLAB_Function : MATLAB Function  TreatAsAtomicUnit=on  SystemSampleTime=T_sampleFFR
  Radians to Degrees : simulink_extras/Transformations/Radians to Degrees
  Rate Transition{,1..5} (6 alike) : RateTransition  OutPortSampleTimeOpt=Inherit
  SaturateAndAlignToComplexS : MATLAB Function  TreatAsAtomicUnit=on
  Scope1 : Scope  NumInputPorts=2
  Scope2 : Scope  NumInputPorts=2
  Scope3 : Scope  NumInputPorts=3
  Scope4 : Scope  NumInputPorts=2
  Scope5 : Scope  NumInputPorts=3
  Three-Phase Sine Generator for Current : spsThreePhaseSineGeneratorLib/Three-Phase Sine Generator  Ts=T_simulation
      settings: LibrarySourceBlock=|
      | sps_lib/Sources/Signal Generator Sources/Three-Phase
      | Sine Generator
  VoltageSupport_pu_GiraldezEtAl : MATLAB Function  TreatAsAtomicUnit=on
  efficiency_applier : MATLAB Function  TreatAsAtomicUnit=on
  p_FCR : Constant  Value=0
  p_pre : Constant  Value=0
  a : PMIOPort  Side=Right
  b : PMIOPort  Port=2  Side=Right
  c : PMIOPort  Port=3  Side=Right
  P_dc : Outport
  wires:
  Complex to Magnitude-Angle/1 -> Gain2/1  "I_rms"
  Demux3/3 -> Controlled Current Source c/1
  efficiency_applier/1(p_bat) -> P_dc/1
  Three-Phase Sine Generator for Current/1 -> Scope4/1, Demux3/1
  Demux3/1 -> Controlled Current Source a/1
  Demux3/2 -> Controlled Current Source b/1
  freq/1 -> [f_sys]
  Max. Injection/Discharge Power/1 -> SaturateAndAlignToComplexS/5(p_max_feedin)  "P_avl_discharge"
  [P_out] -> efficiency_applier/1(p_grid)
  Nominal Voltage/1 -> Divide1/2
  Divide1/1 -> [Voltage_pu], VoltageSupport_pu_GiraldezEtAl/1(v_pu)  "Voltage_pu"
  Max. Absorption/Charge Power/1 -> SaturateAndAlignToComplexS/6(p_max_absorb)  "P_avl_charge"
  SaturateAndAlignToComplexS/2(q_out) -> Scope3/3, Goto4/1  "q_out"
  SaturateAndAlignToComplexS/3(s_out_complex) -> Divide/1, Scope2/1  "s_out_complex"
  [f_sys] -> Three-Phase Sine Generator for Current/3
  Mux:p_pu,q_pu/1 -> Scope5/2
  [phi_i] -> Three-Phase Sine Generator for Current/2
  Gain2/1 -> Three-Phase Sine Generator for Current/1  "I_peak"
  V_LL_rms/1 -> Scope3/1, Memory/1  "V_rms_ASinput"
  Memory/1 -> [V_ac]
  [ppu] -> SaturateAndAlignToComplexS/1(p_PU)
  [ppu] -> Mux:p_pu,q_pu/1  "p_pu"
  [qpu] -> SaturateAndAlignToComplexS/2(q_PU)
  [qpu] -> Mux:p_pu,q_pu/2  "q_pu"
  SaturateAndAlignToComplexS/1(p_out) -> [P_out], Scope3/2  "p_out"
  ICR/1 -> SaturateAndAlignToComplexS/3(ICR)  "ICR"
  ICAR/1 -> SaturateAndAlignToComplexS/4(ICAR)  "ICAR"
  Three-Phase Sine Generator for Current/2 -> Scope4/2
  Complex to Magnitude-Angle/2 -> Radians to Degrees/1  "phi_i_rad"
  Radians to Degrees/1 -> [phi_i]  "phi_i_deg"
  [V_ac] -> Divide/2
  Divide/1 -> Conj/1  "I_complex_conj"
  Conj/1 -> Scope5/3, Scope2/2, Complex to Magnitude-Angle/1  "I_complex"
  Manual Switch3/1 -> Mux1/3, Add/3  "p_FFR1"
  ROCOF_FFR4_MATLAB_Function/1(rocof) -> Rate Transition5/1, FFR4_MATLAB_Function/2(rocof)  "RoCoF_FFR4_100Hz"
  FFR2_MATLAB_Function/1(p_out) -> Rate Transition2/1  "p_FFR2"
  ROCOF_FFR2_MATLAB_Function/1(rocof) -> Rate Transition4/1, FFR2_MATLAB_Function/2(rocof)  "RoCoF_FFR2_100Hz"
  p_FCR/1 -> Add/2, Mux1/2  "p_FCR"
  Manual Switch/1 -> Mux1/6, Add/6  "p_FFR4"
  Constant2/1 -> Manual Switch2/2
  [f_sys] -> FFR3_MATLAB_Function/1(freq)
  Constant3/1 -> Manual Switch3/2
  FFR1_MATLAB_Function/1(p_out) -> Rate Transition3/1  "p_FFR1"
  p_pre/1 -> Add/1, Mux1/1  "p_pre"
  FFR4_MATLAB_Function/1(p_out) -> Rate Transition/1  "p_FFR4"
  [f_sys] -> FFR2_MATLAB_Function/1(freq)
  FFR3_MATLAB_Function/1(p_out) -> Rate Transition1/1  "p_FFR3"
  Constant Time resolution/1 -> ROCOF_FFR2_MATLAB_Function/4(tr)
  Constant/1 -> Manual Switch/2
  [f_sys] -> ROCOF_FFR2_MATLAB_Function/1(freq)
  [Time] -> FFR3_MATLAB_Function/2(time)
  Constant FFR2 Threshold/1 -> ROCOF_FFR2_MATLAB_Function/3(threshold)
  Manual Switch2/1 -> Mux1/4, Add/4  "p_FFR2"
  Manual Switch1/1 -> Mux1/5, Add/5  "p_FFR3"
  Clock/1 -> [Time]
  [f_sys] -> ROCOF_FFR4_MATLAB_Function/1(freq)  "frequency"
  Constant1/1 -> Manual Switch1/2
  [f_sys] -> FFR4_MATLAB_Function/1(freq)
  [Time] -> FFR4_MATLAB_Function/3(time)
  [Time] -> ROCOF_FFR4_MATLAB_Function/2(time)
  [f_sys] -> FFR1_MATLAB_Function/1(freq)
  [Time] -> ROCOF_FFR2_MATLAB_Function/2(time)
  Manual Switch5/1 -> Mux1/7, Add/7  "p_DVS"
  Add/1 -> Mux1/8, [ppu]  "p_pu = p_pre + p_FFR1 + p_FFR2 + p_FFR3 + p_FFR4 + p_DVS"
  [f_sys] -> Scope1/2  "Frequency"
  Mux1/1 -> Scope1/1
  [Voltage_pu] -> Scope5/1
  Constant4/1 -> Manual Switch4/2
  VoltageSupport_pu_GiraldezEtAl/2(q_pu) -> Manual Switch4/1  "q_pu"
  Constant5/1 -> Manual Switch5/2
  VoltageSupport_pu_GiraldezEtAl/1(p_pu) -> Manual Switch5/1  "p_pu"
  Constant6/1 -> efficiency_applier/2(eff)
  [V_ac] -> Divide1/1
  Manual Switch4/1 -> [qpu]  "q_pu"
  Rate Transition/1 -> Manual Switch/1
  Rate Transition1/1 -> Manual Switch1/1
  Rate Transition2/1 -> Manual Switch2/1
  Rate Transition3/1 -> Manual Switch3/1
  Rate Transition4/1 -> ?  "RoCoF_FFR2"
  Rate Transition5/1 -> ?  "RoCoF_FFR4"
  connections:
  Controlled Current Source a/RConn1 -- a/RConn1
  Controlled Current Source c/LConn1 -- Controlled Current Source a/LConn1 -- Controlled Current Source b/LConn1 -- Ground1/LConn1
  Controlled Current Source c/RConn1 -- c/RConn1
  Controlled Current Source b/RConn1 -- b/RConn1

== matlab function SIL_Microgrid/Subsystem_AncillaryServices/Subsystem_BESS/Battery1 ==
  settings: updateMethod=DISCRETE
  data: tr input; States_real output; ProNoise input; Capacity input; I_real input; Rp input; Cp input; States_real input
function States_real = StatReal(tr, ProNoise, Capacity, I_real, Rp, Cp, States_real)
    tao = Rp * Cp;
    Qs = ProNoise(1);
    Qu = ProNoise(2);
    
    A2=exp(-tr/tao);
    A=[1 0;0 A2];  % State transformation matrix
    B1 = -tr/(Capacity*3600);
    B2=Rp*(1-exp(-tr/tao));  
    B=[B1;B2];  % Input control matrix
    States_real = A*States_real + B*I_real + [Qs;Qu];  % 实际过程模拟以 0.1s 更新一次 => Die eigentliche Prozesssimulation wird in 0,1s aktualisiert.

== matlab function SIL_Microgrid/Subsystem_AncillaryServices/Subsystem_FFR_and_VoltageSupport/efficiency_applier ==
  data: p_grid input; p_bat output; eff input
% This function applies an assumed efficiency of the overall BESS to the
% power that is charged or discharged. I.e. increasing the discharge power
% and decreasing the charged power due to losses.
% 
% >Discharge current is defined positive<
%
%##### Input description #####
% p_grid       : active power drawn from or supplied from the grid (in W)
% eff          : efficiency (0...1)
%
%##### Output description #####
% p_bat        : Active Power drawn from of supplied to ideal storage (in W)


function p_bat = efficiency(p_grid, eff)
if p_grid > 0
    p_bat = p_grid / eff;
elseif p_grid < 0
    p_bat = p_grid * eff;
else
    p_bat = 0;
end
end

== matlab function SIL_Microgrid/MATLAB Function ==
  data: p input; s_out_complex output; q input
function s_out_complex = fcn(p,q)
s_out_complex = complex(p,q); 
end

== matlab function SIL_Microgrid/GFM/MATLAB Function1 ==
  data: f output; R_by_X input; V output; SCR input; P_0 input; p_m input; Q_0 input; q_m input; I_RES input; V_offset input
function [f,V] = fcn(R_by_X, SCR, P_0, p_m, Q_0, q_m, I_RES, V_offset)
% Frequency setpoint
f_0 = 50; % Hz
P_b = 10e3; % W
k_p = f_0 * 0.05 / P_b;  % m_p = 5 %

f = f_0 + k_p * (P_0 - p_m);

% Voltage setpoint
V_0 = 400; % V
S_b = 20e3; % VA
k_q = V_0 * 0.1 / S_b; % m_q = 10 %

deltaV_droop = k_q * ( (R_by_X / sqrt(R_by_X^2 + 1)) * (P_0 - p_m) + (1 / sqrt(R_by_X^2 + 1)) * (Q_0 - q_m) );
V_g = V_0 + V_offset + deltaV_droop;
Z_g = V_g^2 / (S_b * SCR);
deltaV_distance = Z_g * I_RES;
V = V_g + deltaV_distance;
end

== matlab function SIL_Microgrid/Subsystem_AncillaryServices/Subsystem_FFR_and_VoltageSupport/SaturateAndAlignToComplexS ==
  data: p_out output; q_out output; p_PU input; q_PU input; s_out_complex output; ICR input; ICAR input; p_max_feedin input; p_max_absorb input
% This function computes the complex power reference for the converter from
% the p.u. values of active and reactive power, respectively, as well as
% the maximum converter power and the maximum available BESS power.
%
% Active power is defined as positive when supplying energy to the grid (=discharging the BESS)
%
%##### Input description #####
% p_PU         : active power reference (in p.u.)
% q_PU         : reactive power reference (in p.u.)
% ICR          : Maximum Converter Power (in VA) (ICR = IBR continuous rating, IBR = Inverter-Based Resources)
% ICAR         : Maximum Converter Power for absorption (in VA) (ICAR = IBR continuous absorption rating)
% p_max_feedin : Maximum available Power from BESS for feedin / discharge BESS (in W)
% p_max_absorb : Maximum available Power from BESS for absorption / charge BESS (in W)
%##### Output description #####
% p_out        : Active Power Reference (in W)
% q_out        : Reactive Power Reference (in var)
% s_out_complex: Complex Power Reference (in VA)

function [p_out,q_out,s_out_complex]  = ComplexApparentPower(p_PU, q_PU, ICR, ICAR, p_max_feedin, p_max_absorb)
% ISR in Watt (ISR = IBR short-term rating) may be added

% Reactive Power
q_out = q_PU*ICR; % q_PU is already saturated to +-0.44, hence no further treatment necessary

% Active Power
if p_PU >= 1              % positive active power, Saturation and Limiting to maximum grid injection / BESS discharge power
    p_out = p_max_feedin; 
elseif p_PU > 0           % positive active power, linear FFR range
    p_out = p_PU * p_max_feedin;
elseif p_PU <= -1         % negative active power, Saturation and Limiting to maximum grid absorption / BESS charge power
    p_out = -abs(p_max_absorb); 
elseif p_PU < 0           % negative active power, linear Voltage support range
    p_out = p_PU * abs(p_max_absorb); % (p_pu is already negative, so multiply with a positive number)
else % p_PU == 0          % zero output power
    p_out = 0;
end

% Complex Power
s_out_complex = complex(p_out,q_out); 
if p_out < 0
    if abs(s_out_complex) > ICAR
        p_out = -sqrt((ICAR^2)-(q_out^2));
    end
else % p_out >= 0
    if abs(s_out_complex) > ICR
        p_out = sqrt((ICR^2)-(q_out^2));
    end
end
    s_out_complex = complex(p_out,q_out); 
end

== matlab function SIL_Microgrid/Subsystem_AncillaryServices/Subsystem_FFR_and_VoltageSupport/VoltageSupport_pu_GiraldezEtAl ==
  data: v_pu input; p_pu output; q_pu output
% This function computes the active and reactive output power in p.u. from
% the measured grid voltage in p.u. according to [Giraldez et al.]

function [p_pu,q_pu] = VoltageSupport(v_pu)

Q_max = 0.44; % in p.u.

if v_pu >= 0.97 && v_pu <= 1.03
    p_pu = 0;
    q_pu = 0;
elseif v_pu > 1.03
    if v_pu < 1.06
        p_pu = 0;
        q_pu = (1.03-v_pu)*(Q_max/0.03);
    elseif v_pu < 1.1
        p_pu = (1.06-v_pu)*(1/0.04);
        q_pu = -Q_max;
    else % v_pu >= 1.1
        p_pu = -1;
        q_pu = -Q_max;
    end
else % v_pu < 0.97
    p_pu = 0;
    if v_pu > 0.94
        q_pu = (0.97-v_pu)*(Q_max/0.03);
    else % v_pu <= 0.94
        q_pu = Q_max;
    end
end
end

== matlab function SIL_Microgrid/Subsystem_AncillaryServices/CalcAvlPwr_MATLAB_Function ==
  data: v_bess input; p_avl_dischg output; soc input; CAPACITY input; p_avl_chg output; C_RATING input
% This function computes the Battery Energy Storage's (BESS') 
% available power for both the discharging and charging case.
% 
%##### Input description #####
% v_bess  : Voltage (V) of the BESS
% soc     : State of Charge (p.u. (1 means full)) of the BESS
% CAPACITY: Capacity (Ah) of the BESS
% C_RATING: C-Rating (p.u.) of the BESS = of the cells
%##### Output description #####
% p_avl_dischg: maximum available discharge power (W) 
% p_avl_chg   : maximum available charge power (W)

function [p_avl_dischg,p_avl_chg] = CalcAvailablePwr(v_bess, soc, CAPACITY, C_RATING) 
%% Constants Definition
DERATING_START_AT_SOC = 0.3;    % Assuming linear derating from SOC=30% downwards and from 70% upwards
P_MAX = C_RATING * CAPACITY * v_bess;  % Maximum BESS power, w/o consideration of SOC.

%% Algorithm for Calculation of available Discharge Power
if soc > DERATING_START_AT_SOC
    p_avl_dischg = P_MAX;
elseif soc > 0
    p_avl_dischg = P_MAX * soc / DERATING_START_AT_SOC;
else 
    p_avl_dischg = 0;
end

%% Algorithm for Calculation of available Charge Power
if soc < (1-DERATING_START_AT_SOC)
    p_avl_chg = P_MAX;
elseif soc < 1
    p_avl_chg = P_MAX * (1-soc) / DERATING_START_AT_SOC;
else
    p_avl_chg = 0;
end
end

== matlab function SIL_Microgrid/Subsystem_AncillaryServices/Subsystem_FFR_and_VoltageSupport/FFR1_MATLAB_Function ==
  data: freq input; p_out output
% This function computes the FFR_1 power output in p.u. based on the
% current measured or observed frequency handed over in Hz. 

function p_out = FFR_1(freq)

fnom = 50;       % 50 Hz
fUF_FFR1 = 49.9; % Minimum: 99.17% of fnom, Maximum: 99.94% of fnom, Default: 99.94% of fnom [IEEE Std 2800-2022], Here: 99.8% of fnom
kUF_FFR1 = 0.01; % Minimum: 1%, Maximum: 5%, Default: 1% [IEEE Std 2800-2022]

if freq<fUF_FFR1
    p_out = (fUF_FFR1 - freq)/(fnom*kUF_FFR1);
else
    p_out = 0;
end
end

== matlab function SIL_Microgrid/Subsystem_AncillaryServices/Subsystem_FFR_and_VoltageSupport/FFR2_MATLAB_Function ==
  data: freq input; p_out output; rocof input
% This function computes the FFR_2 power output in p.u. based on the
% current frequency in Hz and rate of change of frequency (RoCoF) in Hz/s, 
% both handed over as transfer parameters.

function p_out = FFR_2(freq, rocof)

fnom = 50;       % 50 Hz (here just informative)
fUF_FFR2 = 49.7; % Min: 99.17% of fnom, Max: N/A, Default: 99.4% of fnom (used here) [IEEE Std 2800-2022]
kUF_FFR2 = 0.5;  % Min: 0, Max: 5, Default: 0.5 [IEEE Std 2800-2022], (Here: 2.5)

if freq>fUF_FFR2 % idle, i.e. NOT triggered
    p_out = 0;
else % triggered, i.e. freq <= fUF_FFR2
    p_out = -kUF_FFR2 * rocof;
end
end

== matlab function SIL_Microgrid/Subsystem_AncillaryServices/Subsystem_FFR_and_VoltageSupport/FFR4_MATLAB_Function ==
  data: freq input; rocof input; p_out output; time input
% This function computes the FFR_4 power output in p.u. based on passed
% frequency in Hz, rate of change of frequency (RoCoF) in Hz/s and time 
% in seconds. All three are handed over as transfer parameters. 

function p_out = FFR_4(freq, rocof, time)

fnom = 50;           % 50 Hz
dtrigUF_FFR4 = -0.1; % Min: -5.0 Hz/s, Max: 0 Hz/s, Default: -0,5 Hz/s [IEEE Std 2800-2022], Here: -0.1 Hz/s
pT4UF_FFR4 = 0.1;    % Min: 0 p.u., Max: 1 p.u., Default: 0.1 p.u. [IEEE Std 2800-2022], Here: 0.1 p.u.

t_holdFFR = 30;      % [IEEE Std 2800-2022], Annex K.3 (time to hold the support when the trigger is not active any more but frequency has not reached fnom yet)
t_rampFFR = 300;     % [IEEE Std 2800-2022], Annex K.4 (time to ramp down the support after t_holdFFR has been exceeded and fnom has not been reached yet) 

persistent t_trigger;
if isempty(t_trigger)
    t_trigger = -999;
end

if freq<=fnom
    if rocof<=dtrigUF_FFR4 % TRIGGER  (greater/less sign swapped compared to [IEEE Std 2800-2022])
        t_trigger = time; % may be set several times, stores the last trigger event
        p_out = pT4UF_FFR4;
    else % (rocof > dtrigUF_FFR4) AND freq <= fnom: continue operation during t_holdFFR and derate for t_rampFFR
        if (time - t_trigger) <= t_holdFFR % continue
            p_out = pT4UF_FFR4; 
        elseif (time - t_trigger) <= (t_holdFFR+t_rampFFR) % derate
            p_out = pT4UF_FFR4*(1-(time - t_trigger - t_holdFFR) / (t_rampFFR)); 
        else % time elapsed since last trigger event > (t_holdFFR+t_rampFFR)
            p_out = 0;
        end
    end
else % freq>fnom
    t_trigger = -999; % reset trigger
    p_out = 0; 
end
end

== matlab function SIL_Microgrid/Subsystem_AncillaryServices/Subsystem_FFR_and_VoltageSupport/FFR3_MATLAB_Function ==
  data: freq input; p_out output; time input
% This function computes the FFR_3 power output in p.u. based on the
% current frequency in Hz and time in seconds. Both are handed over as
% transfer parameters.

function p_out = FFR_3(freq, time)

fnom = 50;            % 50 Hz
fUF_FFR3 = 49.7;      % basic support threshold (where pT3UF_FFR3 is used)
fUF_FFR3_1 = 49.65;   % 1st extra support threshold (where pT3UF_FFR3_1 is used)
fUF_FFR3_2 = 49.6;    % 2nd extra support threshold (where pT3UF_FFR3_2 is used)
pT3UF_FFR3 = 0.33;    % basic support power
pT3UF_FFR3_1 = 0.66;  % 1st extra support power
pT3UF_FFR3_2 = 1;     % 2nd extra support power
t_holdFFR = 30;       % [IEEE Std 2800-2022], Annex K.3 (time to hold the support when the trigger is not active any more but frequency has not reached fnom yet)
t_rampFFR = 300;      % [IEEE Std 2800-2022], Annex K.4 (time to ramp down the support after t_holdFFR has been exceeded and fnom has not been reached yet) 

persistent t_trigger;
if isempty(t_trigger)
    t_trigger = -999;
end

if freq<=fnom
    if freq>fUF_FFR3_1     % freq=(fUF_FFR3_1 , fUF_FFR3]
        P = pT3UF_FFR3;
    elseif freq>fUF_FFR3_2 % freq=(fUF_FFR3_2 , fUF_FFR3_1]
        P = pT3UF_FFR3_1;
    elseif freq>=47.5      % freq=[47.5 , fUF_FFR3_2]
        P = pT3UF_FFR3_2;
    else                   % freq<47.5 Hz
        P = 0;
    end

    if freq<fUF_FFR3 % Trigger
        t_trigger = time; % may be set several times, stores last trigger event
        p_out = P;
    else % fUF_FFR3 <= freq <= fnom: continue operation during t_holdFFR and derate for t_rampFFR
        if (time - t_trigger) <= t_holdFFR % hold
            p_out = P;
        elseif (time - t_trigger) <= (t_holdFFR+t_rampFFR) % derate
            p_out = P*(1-(time - t_trigger - t_holdFFR) / (t_rampFFR));
        else % time elapsed since last trigger event > (t_holdFFR+t_rampFFR)
            p_out = 0;
        end
    end

else % freq>fnom
    t_trigger = -999; % reset trigger
    p_out = 0;
end
end
